simulink model "MdSWReqChk"  (R2024b)
settings: Solver=FixedStepDiscrete  StartTime=0.0  StopTime=10.0  FixedStep=0.01  RelTol=1e-3
undefined symbols (not defined in the file or in its folder): ChkBsyBitArray4s, ChkBsyBitArray6s7s, KeSMSAutoEZEFwdBkwdPosEna_Val, KeSMSuButtonLongPressedThrshldTm_Val, KeSMSuMdNum4s_Val, KeSMSuMdNum6s7s_Val, SetBsyBitArray4s, SetEnBitArray4s
libraries: simulink x16, RspLib x14
(part 2 of 3)

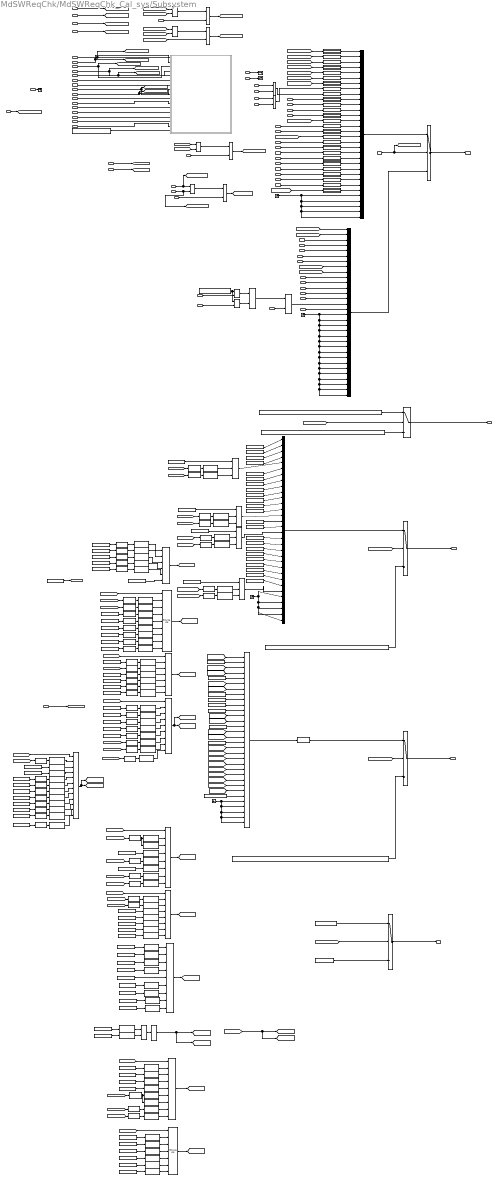
== system MdSWReqChk/MdSWReqChk_Cal_sys/Subsystem ==
  note: 0000 0010 1100 1101 1110 0000 0111 1000
  note: 2023.12.28 迎宾向后，条件改为或
  note: bug542961
  note: 符号方向反了，<= 改为>=
  note: 2023.8.1 CR401790 增加模式21-26的请求
  note: VIPR
  note: RcvyR
  note: VIPR
  note: LugL
  note: LugL
  note: LugR
  note: LugL
  note: LugL
  note: LugL
  note: LugR
  note: VIPR
  note: Md57
  note: Md57
  note: Md57
  note: LugR
  note: bedr
  acsEntyMdReq_Val_read : Inport
  acsExtMdReq_Val_read : Inport  Port=2
  AllLugMdReq_Val_read : Inport  Port=3
  AllVipMdReq_Val_read : Inport  Port=4
  EZE4sLtMdReq_Val_read : Inport  Port=5
  EZE4sRtMdReq_Val_read : Inport  Port=6
  EZQ4sLtMdReq_Val_read : Inport  Port=7
  EZQ4sRtMdReq_Val_read : Inport  Port=8
  IntimacyRtMdReq_Val_read : Inport  Port=9
  INTMMdReq_Val_read : Inport  Port=10
  LfFamlyReq_Val_read : Inport  Port=11
  LfLyMdReq_Val_read : Inport  Port=12
  LgrstCloseLtMdReq_Val_read : Inport  Port=13
  LgrstCloseRtMdReq_Val_read : Inport  Port=14
  LgrstOpenLtMdReq_Val_read : Inport  Port=15
  LgrstOpenRtMdReq_Val_read : Inport  Port=16
  LtLugMdReq_Val_read : Inport  Port=17
  LtRcvyMdReq_Val_read : Inport  Port=18
  LtVipMdReq_Val_read : Inport  Port=19
  LugMdLtAvl_Val_read : Inport  Port=20
  LugMdRtAvl_Val_read : Inport  Port=21
  MdSWIntSrc_R_Val_read : Inport  Port=22
  RtFamlyMdReq_Val_read : Inport  Port=23
  RtLugMdReq_Val_read : Inport  Port=24
  RtLyMdReq_Val_read : Inport  Port=25
  RtRcvyMdReq_Val_read : Inport  Port=26
  RtVipMdReq_Val_read : Inport  Port=27
  StNumFlg_Is4s_read : Inport  Port=28
  StNumFlg_Is6s_read : Inport  Port=29
  StNumFlg_Is6s7s_read : Inport  Port=30
  StNumFlg_Is7s_read : Inport  Port=31
  SwIntAcsEnty_Val_read : Inport  Port=32
  SwIntAcsExt_Val_read : Inport  Port=33
  SwIntAllLug_Val_read : Inport  Port=34
  SwIntLfRcvy_Val_read : Inport  Port=35
  SwIntLfVip_Val_read : Inport  Port=36
  SwIntRtRcvy_Val_read : Inport  Port=37
  SwIntRtVip_Val_read : Inport  Port=38
  VipMdLtAvl_Val_read : Inport  Port=39
  VipMdRtAvl_Val_read : Inport  Port=40
  WelcomeBkwdMdReq_Val_read : Inport  Port=41
  WelcomeFwdMdReq_Val_read : Inport  Port=42
  modestate32 : Inport  Port=43
  IfVeSMSuSecRwLtStFrwdBkwdPos_Val_read : Inport  Port=44
  IfVeSMSuSecRwRtStFrwdBkwdPos_Val_read : Inport  Port=45
  Md27Req_Val_read : Inport  Port=46
  Md28Req_Val_read : Inport  Port=47
  Md30Req_Val_read : Inport  Port=48
  Md31Req_Val_read : Inport  Port=49
  Md32Req_Val_read : Inport  Port=50
  Md53Req_Val_read : Inport  Port=51
  Md29Req_Val_read : Inport  Port=52
  VipExitMdLtAvl_Val_read : Inport  Port=53
  VipExitMdRtAvl_Val_read : Inport  Port=54
  Md56Req_Val_read : Inport  Port=55
  Md57Req_Val_read : Inport  Port=56
  Md58Req_Val_read : Inport  Port=57
  Md62Req_Val_read : Inport  Port=58
  Md61Req_Val_read : Inport  Port=59
  Md61MemReq_Val_read : Inport  Port=60
  Md62MemReq_Val_read : Inport  Port=61
  BigBedAllMdReq_Val_read : Inport  Port=62
  BigBedLMdAvl_Val_read : Inport  Port=63
  BigBedLtMdReq_Val_read : Inport  Port=64
  BigBedRMdAvl_Val_read : Inport  Port=65
  BigBedRtMdReq_Val_read : Inport  Port=66
  Bitwise Operator{,1,6,15} (4 alike) : simulink/Logic and Bit Operations/Bitwise Operator  logicop=OR  UseBitMask=off  NumInputPorts=3  BitMask=bin2dec('11011001')  BitMaskRealWorld=Stored Integer
  Bitwise Operator10 : simulink/Logic and Bit Operations/Bitwise Operator  logicop=OR  UseBitMask=off  NumInputPorts=7  BitMask=bin2dec('11011001')  BitMaskRealWorld=Stored Integer
  Bitwise Operator{2,8..9,11} (4 alike) : simulink/Logic and Bit Operations/Bitwise Operator  logicop=OR  UseBitMask=off  NumInputPorts=9  BitMask=bin2dec('11011001')  BitMaskRealWorld=Stored Integer
  Bitwise Operator12 : simulink/Logic and Bit Operations/Bitwise Operator  logicop=OR  UseBitMask=off  NumInputPorts=7  BitMask=bin2dec('11011001')  BitMaskRealWorld=Stored Integer
  Bitwise Operator13 : simulink/Logic and Bit Operations/Bitwise Operator  logicop=OR  UseBitMask=off  NumInputPorts=2  BitMask=bin2dec('11011001')  BitMaskRealWorld=Stored Integer
  Bitwise Operator14 : simulink/Logic and Bit Operations/Bitwise Operator  logicop=NOT  UseBitMask=off  BitMask=bin2dec('11011001')  BitMaskRealWorld=Stored Integer
  Bitwise Operator3 : simulink/Logic and Bit Operations/Bitwise Operator  logicop=OR  UseBitMask=off  NumInputPorts=12  BitMask=bin2dec('11011001')  BitMaskRealWorld=Stored Integer
  Bitwise Operator4 : simulink/Logic and Bit Operations/Bitwise Operator  logicop=OR  UseBitMask=off  NumInputPorts=8  BitMask=bin2dec('11011001')  BitMaskRealWorld=Stored Integer
  Bitwise Operator5 : simulink/Logic and Bit Operations/Bitwise Operator  logicop=OR  UseBitMask=off  NumInputPorts=8  BitMask=bin2dec('11011001')  BitMaskRealWorld=Stored Integer
  Bitwise Operator7 : simulink/Logic and Bit Operations/Bitwise Operator  logicop=OR  UseBitMask=off  NumInputPorts=6  BitMask=bin2dec('11011001')  BitMaskRealWorld=Stored Integer
  Constant : Constant  Value=ChkBsyBitArray6s7s  OutDataTypeStr=uint32
  Constant1 : Constant  Value=ChkBsyBitArray4s  OutDataTypeStr=uint32
  Constant10 : Constant  Value=268435456  OutDataTypeStr=uint32
  Constant101 : Constant  Value=0xffffffff  OutDataTypeStr=uint32
  Constant{19..20,24..25,39..44,47,50..55,57..60,62..66,68..92,94,102} (53 alike) : Constant  OutDataTypeStr=uint32
  Constant{11..18} (8 alike) : Constant  Value=4294967295  OutDataTypeStr=uint32
  Constant2 : Constant  Value=SetEnBitArray4s  OutDataTypeStr=uint32
  Constant21 : Constant  Value=1048576  OutDataTypeStr=uint32
  Constant22 : Constant  Value=2097152  OutDataTypeStr=uint32
  Constant{23,45..46,48..49,61,67,93} (8 alike) : Constant  Value=0  OutDataTypeStr=uint32
  Constant26 : Constant  Value=8  OutDataTypeStr=uint32
  Constant27 : Constant  Value=512  OutDataTypeStr=uint32
  Constant28 : Constant  Value=2048  OutDataTypeStr=uint32
  Constant29 : Constant  Value=2  OutDataTypeStr=uint32
  Constant3 : Constant  Value=67108864  OutDataTypeStr=uint32
  Constant30 : Constant  Value=1024  OutDataTypeStr=uint32
  Constant31 : Constant  Value=4096  OutDataTypeStr=uint32
  Constant32 : Constant  Value=64  OutDataTypeStr=uint32
  Constant33 : Constant  Value=32  OutDataTypeStr=uint32
  Constant34 : Constant  Value=16  OutDataTypeStr=uint32
  Constant35 : Constant  Value=524288  OutDataTypeStr=uint32
  Constant36 : Constant  Value=128  OutDataTypeStr=uint32
  Constant37 : Constant  Value=256  OutDataTypeStr=uint32
  Constant38 : Constant  Value=4  OutDataTypeStr=uint32
  Constant4 : Constant  Value=134217728  OutDataTypeStr=uint32
  Constant5 : Constant  Value=536870912  OutDataTypeStr=uint32
  Constant56 : Constant  Value=16777216  OutDataTypeStr=uint32
  Constant6 : Constant  Value=1073741824  OutDataTypeStr=uint32
  Constant7 : Constant  Value=SetBsyBitArray4s  OutDataTypeStr=uint32
  Constant8 : Constant  Value=2147483648  OutDataTypeStr=uint32
  Constant9 : Constant  Value=131072  OutDataTypeStr=uint32
  Constant95 : Constant  Value=8192  OutDataTypeStr=uint32
  Constant96 : Constant  Value=16384  OutDataTypeStr=uint32
  Constant98 : Constant  Value=32768  OutDataTypeStr=uint32
  Data Type Conversion{,1..10,12..51,53..54} (53 alike) : DataTypeConversion  OutDataTypeStr=uint32  SaturateOnIntegerOverflow=off  RndMeth=Floor
  Data Type Conversion11 : DataTypeConversion  SaturateOnIntegerOverflow=off  RndMeth=Floor
  Ground{,1..3} (4 alike) : Ground
  Logical Operator{,2,4,6,8..10} (7 alike) : Logic  Operator=OR  AllPortsSameDT=off  OutDataTypeStr=boolean
  Logical Operator{1,3,5,7,11} (5 alike) : Logic  AllPortsSameDT=off  OutDataTypeStr=boolean
  Mux{,1..3} (4 alike) : Mux  Inputs=32
  NotUsedMode : Constant  Value=47046776  OutDataTypeStr=uint32
  PA_KeSMSAutoEZEFwdBkwdPosEna_Val : Constant  Value=KeSMSAutoEZEFwdBkwdPosEna_Val
  PA_KeSMSuButtonLongPressedThrshldTm_Val : Constant  Value=KeSMSuButtonLongPressedThrshldTm_Val
  PA_KeSMSuMdNum4s_Val : Constant  Value=KeSMSuMdNum4s_Val
  PA_KeSMSuMdNum6s7s_Val : Constant  Value=KeSMSuMdNum6s7s_Val
  Relational Operator : RelationalOperator  OutDataTypeStr=boolean  RndMeth=Simplest  InputSameDT=off
  Relational Operator1 : RelationalOperator  OutDataTypeStr=boolean  RndMeth=Simplest  InputSameDT=off
  ReqTrig : Subsystem
  ReqTrig1 : Subsystem
  ReqTrig10 : Subsystem
  ReqTrig11 : Subsystem
  ReqTrig12 : Subsystem
  ReqTrig13 : Subsystem
  ReqTrig14 : Subsystem
  ReqTrig15 : Subsystem
  ReqTrig16 : Subsystem
  ReqTrig17 : Subsystem
  ReqTrig18 : Subsystem
  ReqTrig19 : Subsystem
  ReqTrig2 : Subsystem
  ReqTrig20 : Subsystem
  ReqTrig21 : Subsystem
  ReqTrig22 : Subsystem
  ReqTrig23 : Subsystem
  ReqTrig24 : Subsystem
  ReqTrig25 : Subsystem
  ReqTrig26 : Subsystem
  ReqTrig3 : Subsystem
  ReqTrig4 : Subsystem
  ReqTrig5 : Subsystem
  ReqTrig6 : Subsystem
  ReqTrig7 : Subsystem
  ReqTrig8 : Subsystem
  ReqTrig9 : Subsystem
  Shift Arithmetic{,27,44,52} (4 alike) : ArithShift  BitShiftNumber=9  BitShiftDirection=Left
  Shift Arithmetic{1,8..9,20,45,55,58} (7 alike) : ArithShift  BitShiftNumber=11  BitShiftDirection=Left
  Shift Arithmetic10 : ArithShift  BitShiftNumber=26  BitShiftDirection=Left
  Shift Arithmetic{11,26,36,39} (4 alike) : ArithShift  BitShiftNumber=27  BitShiftDirection=Left
  Shift Arithmetic12 : ArithShift  BitShiftNumber=29  BitShiftDirection=Left
  Shift Arithmetic13 : ArithShift  BitShiftNumber=30  BitShiftDirection=Left
  Shift Arithmetic{14,28,33,50} (4 alike) : ArithShift  BitShiftNumber=31  BitShiftDirection=Left
  Shift Arithmetic{3,15,23..24,47,57} (6 alike) : ArithShift  BitShiftNumber=8  BitShiftDirection=Left
  Shift Arithmetic16 : ArithShift  BitShiftDirection=Left
  Shift Arithmetic17 : ArithShift  BitShiftNumber=1  BitShiftDirection=Left
  Shift Arithmetic18 : ArithShift  BitShiftNumber=2  BitShiftDirection=Left
  Shift Arithmetic19 : ArithShift  BitShiftNumber=24  BitShiftDirection=Left
  Shift Arithmetic{2,5,22,25,31,46,51} (7 alike) : ArithShift  BitShiftNumber=7  BitShiftDirection=Left
  Shift Arithmetic{21,35,38,40,56} (5 alike) : ArithShift  BitShiftNumber=17  BitShiftDirection=Left
  Shift Arithmetic29 : ArithShift  BitShiftNumber=26  BitShiftDirection=Left
  Shift Arithmetic30 : ArithShift  BitShiftNumber=28  BitShiftDirection=Left
  Shift Arithmetic32 : ArithShift  BitShiftNumber=10  BitShiftDirection=Left
  Shift Arithmetic34 : ArithShift  BitShiftNumber=26  BitShiftDirection=Left
  Shift Arithmetic37 : ArithShift  BitShiftNumber=13  BitShiftDirection=Left
  Shift Arithmetic{4,6..7,42,54,59} (6 alike) : ArithShift  BitShiftNumber=12  BitShiftDirection=Left
  Shift Arithmetic41 : ArithShift  BitShiftNumber=1  BitShiftDirection=Left
  Shift Arithmetic43 : ArithShift  BitShiftNumber=10  BitShiftDirection=Left
  Shift Arithmetic48 : ArithShift  BitShiftNumber=29  BitShiftDirection=Left
  Shift Arithmetic49 : ArithShift  BitShiftNumber=30  BitShiftDirection=Left
  Shift Arithmetic53 : ArithShift  BitShiftNumber=10  BitShiftDirection=Left
  Shift Arithmetic{60,62,64,66,68,70,72,74} (8 alike) : ArithShift  BitShiftNumber=20  BitShiftDirection=Left
  Shift Arithmetic{61,63,65,67,69,71,73,75} (8 alike) : ArithShift  BitShiftNumber=21  BitShiftDirection=Left
  Shift Arithmetic76 : ArithShift  BitShiftNumber=29  BitShiftDirection=Left
  Shift Arithmetic77 : ArithShift  BitShiftNumber=30  BitShiftDirection=Left
  Shift Arithmetic78 : ArithShift  BitShiftNumber=14  BitShiftDirection=Left
  Shift Arithmetic80 : ArithShift  BitShiftNumber=14  BitShiftDirection=Left
  Shift Arithmetic81 : ArithShift  BitShiftNumber=13  BitShiftDirection=Left
  Subsystem : Subsystem  Commented=on
  Switch{,1..4} (5 alike) : Switch  Criteria=u2 > Threshold  SaturateOnIntegerOverflow=off  InputSameDT=off
  Terminator : Terminator
  Terminator1 : Terminator
  Terminator_28 : Terminator
  VIPR : ArithShift  BitShiftNumber=11  BitShiftDirection=Left
  VIPR1 : ArithShift  BitShiftNumber=27  BitShiftDirection=Left
  VIPR2 : ArithShift  BitShiftNumber=28  BitShiftDirection=Left
  ChkBsyBitArray_Val_write : Outport  VectorParamsAs1DForOutWhenUnconnected=off
      settings: EnsureOutportIsVirtual=on
  MdReqArray_Val_write : Outport  Port=2  VectorParamsAs1DForOutWhenUnconnected=off
      settings: EnsureOutportIsVirtual=on
  SetBsyBitArray_Val_write : Outport  Port=3  VectorParamsAs1DForOutWhenUnconnected=off
      settings: EnsureOutportIsVirtual=on
  SetEnBitArray_Val_write : Outport  Port=4  VectorParamsAs1DForOutWhenUnconnected=off
      settings: EnsureOutportIsVirtual=on
  VeSMSuMdNum_Val_write : Outport  Port=5  VectorParamsAs1DForOutWhenUnconnected=off
      settings: EnsureOutportIsVirtual=on
  wires:
  StNumFlg_Is4s_read/1 -> Terminator_28/1
  StNumFlg_Is7s_read/1 -> [is7s]
  PA_KeSMSuButtonLongPressedThrshldTm_Val/1 -> Subsystem/17(KeSMSuButtonLongPressedThrshldTm_Val)
  StNumFlg_Is6s_read/1 -> [Is6s]
  modestate32/1 -> Subsystem/7(modestate32_Val_read)
  acsEntyMdReq_Val_read/1 -> [EZEReq], Subsystem/1(acsEntyMdReq_Val_read)
  AllLugMdReq_Val_read/1 -> [AllLugReq], Subsystem/3(AllLugMdReq_Val_read)
  acsExtMdReq_Val_read/1 -> [EZQReq], Subsystem/2(acsExtMdReq_Val_read)
  MdSWIntSrc_R_Val_read/1 -> Subsystem/6(MdSWIntSrc_R_Val_read)
  LtVipMdReq_Val_read/1 -> [LtVIPReq], Subsystem/5(LtVipMdReq_Val_read)
  LtRcvyMdReq_Val_read/1 -> [LtRcvyReq], Subsystem/4(LtRcvyMdReq_Val_read)
  RtRcvyMdReq_Val_read/1 -> [RtRcvyReq], Subsystem/8(RtRcvyMdReq_Val_read)
  RtVipMdReq_Val_read/1 -> [RtVIPReq], Subsystem/9(RtVipMdReq_Val_read)
  SwIntAcsEnty_Val_read/1 -> Subsystem/10(SwIntAcsEnty_Val_read)
  SwIntAcsExt_Val_read/1 -> Subsystem/11(SwIntAcsExt_Val_read)
  SwIntLfRcvy_Val_read/1 -> Subsystem/12(SwIntLfRcvy_Val_read)
  SwIntLfVip_Val_read/1 -> Subsystem/13(SwIntLfVip_Val_read)
  SwIntRtVip_Val_read/1 -> Subsystem/15(SwIntRtVip_Val_read)
  SwIntAllLug_Val_read/1 -> Subsystem/16(SwIntAllLug_Val_read)
  SwIntRtRcvy_Val_read/1 -> Subsystem/14(SwIntRtRcvy_Val_read)
  [EZEReq] -> ReqTrig/1(Req)
  [EZQReq] -> ReqTrig1/1(Req)
  [LtVIPReq] -> ReqTrig2/1(Req)
  [RtVIPReq] -> ReqTrig3/1(Req)
  VipMdLtAvl_Val_read/1 -> [VipLtAvl]
  VipMdRtAvl_Val_read/1 -> [VipRtAvl]
  [VipLtAvl] -> Logical Operator/1
  [VipRtAvl] -> Logical Operator/2
  Logical Operator/1 -> Logical Operator1/1
  AllVipMdReq_Val_read/1 -> Logical Operator1/2
  Logical Operator1/1 -> [AllVipReq]
  [AllVipReq] -> ReqTrig4/1(Req)
  [LtRcvyReq] -> ReqTrig5/1(Req)
  [RtRcvyReq] -> ReqTrig6/1(Req)
  INTMMdReq_Val_read/1 -> ReqTrig9/1(Req)
  IntimacyRtMdReq_Val_read/1 -> ReqTrig10/1(Req)
  LtLugMdReq_Val_read/1 -> ReqTrig11/1(Req)
  RtLugMdReq_Val_read/1 -> ReqTrig12/1(Req)
  Logical Operator3/1 -> [AllLugReqComfirm]
  [AllLugReq] -> Logical Operator3/2
  Logical Operator2/1 -> Logical Operator3/1
  LugMdLtAvl_Val_read/1 -> [LugLtAvl]
  LugMdRtAvl_Val_read/1 -> [LugRtAvl]
  [LugLtAvl] -> Logical Operator2/1
  [LugRtAvl] -> Logical Operator2/2
  [AllLugReqComfirm] -> ReqTrig13/1(Req)
  Switch/1 -> MdReqArray_Val_write/1
  StNumFlg_Is6s7s_read/1 -> [Is6s7s], Switch/2
  Mux/1 -> Switch/1
  [LtVIPReq] -> Mux1/1
  [LtRcvyReq] -> Mux1/2
  LfLyMdReq_Val_read/1 -> Mux1/3
  LgrstOpenLtMdReq_Val_read/1 -> Mux1/4
  LgrstCloseLtMdReq_Val_read/1 -> Mux1/5
  [RtVIPReq] -> Mux1/8
  [RtRcvyReq] -> Mux1/9
  RtLyMdReq_Val_read/1 -> Mux1/10
  LgrstOpenRtMdReq_Val_read/1 -> Mux1/11
  LgrstCloseRtMdReq_Val_read/1 -> Mux1/12
  EZE4sRtMdReq_Val_read/1 -> Mux1/13
  EZQ4sRtMdReq_Val_read/1 -> Mux1/14
  WelcomeFwdMdReq_Val_read/1 -> Mux1/16
  Ground1/1 -> Mux1/27, Mux1/28, Mux1/32, Mux1/31, Mux1/30, Mux1/29, Mux1/26, Mux1/25, Mux1/24, Mux1/23, Mux1/22, Mux1/21, Mux1/20, Mux1/19, Mux1/18, Mux1/17
  Mux1/1 -> Switch/3
  [Is6s7s] -> Switch1/2
  Switch1/1 -> ChkBsyBitArray_Val_write/1
  Constant/1 -> Switch1/1
  Constant1/1 -> Switch1/3
  Constant2/1 -> Switch2/3
  [Is6s7s] -> Switch2/2
  Constant33/1 -> Mux2/9
  Mux2/1 -> Switch2/1  "SetEnBitArray"
  Data Type Conversion/1 -> Shift Arithmetic/1
  Constant37/1 -> Mux2/13
  Constant39/1 -> Mux2/1
  [VipRtAvl] -> Data Type Conversion1/1
  Constant28/1 -> Mux2/4
  Constant26/1 -> Mux2/2
  Bitwise Operator/1 -> Mux2/5
  Constant32/1 -> Mux2/8
  Constant30/1 -> Mux2/6
  Bitwise Operator1/1 -> Mux2/14
  Constant35/1 -> Mux2/11
  [VipLtAvl] -> Data Type Conversion/1
  Constant31/1 -> Mux2/7
  Constant34/1 -> Mux2/10
  Constant36/1 -> Mux2/12
  Constant29/1 -> Bitwise Operator/1
  [LugLtAvl] -> Data Type Conversion2/1
  Shift Arithmetic/1 -> Bitwise Operator/2
  Constant27/1 -> Mux2/3
  Data Type Conversion1/1 -> Shift Arithmetic1/1
  Constant38/1 -> Bitwise Operator1/1
  Shift Arithmetic1/1 -> Bitwise Operator/3
  Data Type Conversion2/1 -> Shift Arithmetic2/1
  Shift Arithmetic2/1 -> Bitwise Operator1/2
  [LugRtAvl] -> Data Type Conversion3/1
  Data Type Conversion3/1 -> Shift Arithmetic3/1
  Shift Arithmetic3/1 -> Bitwise Operator1/3
  Switch2/1 -> SetEnBitArray_Val_write/1
  Switch3/1 -> SetBsyBitArray_Val_write/1
  [Is6s7s] -> Switch3/2
  Constant7/1 -> Switch3/3
  Constant12/1 -> Mux3/5
  Constant16/1 -> Mux3/10
  Data Type Conversion11/1 -> Switch3/1  "SetBsyBitArray"
  Constant15/1 -> Mux3/9
  Constant14/1 -> Mux3/8
  [BsyBitEZE] -> Mux3/1
  [RghtBsyBitLug] -> Mux3/13
  Constant17/1 -> Mux3/11
  [RghtBsyBitRcvy] -> Mux3/7
  Constant11/1 -> Mux3/2
  [LftBsyBitVIP] -> Mux3/3
  [LftBsyBitLug] -> Mux3/12
  Mux3/1 -> Data Type Conversion11/1
  [RghtBsyBitVIP] -> Mux3/4
  [LftBsyBitRcvy] -> Mux3/6
  [is7s] -> Data Type Conversion5/1
  Shift Arithmetic8/1 -> Bitwise Operator4/3
  [BsyAll] -> Bitwise Operator4/1
  [is7s] -> Data Type Conversion7/1
  [is7s] -> Data Type Conversion6/1
  Shift Arithmetic9/1 -> Bitwise Operator5/2
  [BsyAll] -> Bitwise Operator5/1
  Bitwise Operator3/1 -> [RghtBsyBitVIP], [VIPRExitBsyBit]
  Data Type Conversion7/1 -> Shift Arithmetic9/1
  Bitwise Operator4/1 -> [LftBsyBitLug]
  Shift Arithmetic6/1 -> Bitwise Operator4/2
  Data Type Conversion5/1 -> Shift Arithmetic5/1
  [BsyAll] -> Bitwise Operator2/1
  Data Type Conversion6/1 -> Shift Arithmetic8/1, Shift Arithmetic6/1
  Bitwise Operator5/1 -> [RghtBsyBitLug]
  Shift Arithmetic5/1 -> Bitwise Operator3/2
  Bitwise Operator2/1 -> [LftBsyBitVIP], [VIPLExitBsyBit]
  [BsyAll] -> Bitwise Operator3/1
  [Is6s7s] -> Switch4/2
  PA_KeSMSuMdNum4s_Val/1 -> Switch4/3
  PA_KeSMSuMdNum6s7s_Val/1 -> Switch4/1  "SetBsyBitArray"
  Switch4/1 -> VeSMSuMdNum_Val_write/1
  PA_KeSMSAutoEZEFwdBkwdPosEna_Val/1 -> Relational Operator1/1, Relational Operator/1
  IfVeSMSuSecRwLtStFrwdBkwdPos_Val_read/1 -> Relational Operator/2
  IfVeSMSuSecRwRtStFrwdBkwdPos_Val_read/1 -> Relational Operator1/2
  Relational Operator/1 -> Logical Operator4/1
  Relational Operator1/1 -> Logical Operator4/2
  Logical Operator5/1 -> Mux1/15
  WelcomeBkwdMdReq_Val_read/1 -> Logical Operator5/2
  Logical Operator4/1 -> Logical Operator5/1
  Md27Req_Val_read/1 -> ReqTrig14/1(Req)
  Md28Req_Val_read/1 -> ReqTrig15/1(Req)
  Constant3/1 -> Mux2/15
  Constant4/1 -> Mux2/16
  [Md29Req] -> ReqTrig16/1(Req)
  Md32Req_Val_read/1 -> ReqTrig19/1(Req)
  Md53Req_Val_read/1 -> ReqTrig20/1(Req)
  Constant5/1 -> Mux2/18
  Constant6/1 -> Mux2/19
  Constant8/1 -> Mux2/20
  Bitwise Operator6/1 -> Mux2/17
  Constant10/1 -> Bitwise Operator6/1
  Shift Arithmetic10/1 -> Bitwise Operator6/2
  Data Type Conversion8/1 -> Shift Arithmetic10/1
  [VIPLExittAvl] -> Data Type Conversion8/1
  [VIPRExittAvl] -> Data Type Conversion9/1
  Data Type Conversion9/1 -> Shift Arithmetic11/1
  Shift Arithmetic11/1 -> Bitwise Operator6/3
  Constant13/1 -> Mux3/14
  [VIPLExitBsyBit] -> Mux3/15
  [VIPRExitBsyBit] -> Mux3/16
  Constant18/1 -> Mux3/17
  [BsyBitThdExpandL] -> Mux3/20
  [BsyBitThdExpandR] -> Mux3/21
  Constant41/1 -> Shift Arithmetic12/1
  Constant43/1 -> Shift Arithmetic13/1
  Shift Arithmetic12/1 -> Bitwise Operator3/3
  Shift Arithmetic13/1 -> Bitwise Operator3/4
  Shift Arithmetic14/1 -> Bitwise Operator4/4
  Constant44/1 -> Shift Arithmetic14/1
  [BsyBitPass] -> Mux3/18
  [BsyBitPass] -> Mux3/19
  [BsyAll] -> Bitwise Operator9/1
  Shift Arithmetic22/1 -> Bitwise Operator9/2
  Data Type Conversion12/1 -> Shift Arithmetic22/1
  Bitwise Operator9/1 -> [RghtBsyBitRcvy]
  VipExitMdLtAvl_Val_read/1 -> [VIPLExittAvl]
  VipExitMdRtAvl_Val_read/1 -> [VIPRExittAvl]
  [VIPRExittAvl] -> Logical Operator6/2
  [VIPLExittAvl] -> Logical Operator6/1
  Logical Operator6/1 -> Logical Operator7/1
  Md29Req_Val_read/1 -> Logical Operator7/2
  Logical Operator7/1 -> [Md29Req]
  [is7s] -> Data Type Conversion12/1
  Bitwise Operator10/1 -> [LftBsyBitRcvy]
  [BsyAll] -> Bitwise Operator10/1
  Constant23/1 -> Data Type Conversion13/1
  Data Type Conversion13/1 -> Shift Arithmetic23/1
  Shift Arithmetic23/1 -> Bitwise Operator10/2
  Shift Arithmetic24/1 -> Bitwise Operator9/3  "LugR"
  Data Type Conversion14/1 -> Shift Arithmetic24/1
  [is7s] -> Data Type Conversion14/1
  Shift Arithmetic25/1 -> Bitwise Operator10/3
  Data Type Conversion15/1 -> Shift Arithmetic25/1
  [is7s] -> Data Type Conversion15/1
  Md56Req_Val_read/1 -> ReqTrig21/1(Req)
  [BsyBitBigFourSt] -> Mux3/22
  Md30Req_Val_read/1 -> ReqTrig17/1(Req)
  Md31Req_Val_read/1 -> ReqTrig18/1(Req)
  Constant51/1 -> VIPR/1
  Constant47/1 -> Data Type Conversion16/1
  Data Type Conversion16/1 -> Shift Arithmetic16/1
  Constant48/1 -> Data Type Conversion17/1
  Data Type Conversion17/1 -> Shift Arithmetic17/1
  Data Type Conversion18/1 -> Shift Arithmetic18/1
  Constant49/1 -> Data Type Conversion18/1
  Bitwise Operator7/1 -> [BsyAll]
  Constant50/1 -> Data Type Conversion19/1
  Data Type Conversion19/1 -> Shift Arithmetic19/1
  Constant52/1 -> Data Type Conversion20/1
  Data Type Conversion20/1 -> Shift Arithmetic20/1
  Data Type Conversion21/1 -> Shift Arithmetic21/1
  Constant53/1 -> Data Type Conversion21/1
  Constant54/1 -> Data Type Conversion22/1
  Data Type Conversion22/1 -> Shift Arithmetic26/1
  Shift Arithmetic20/1 -> Bitwise Operator9/4  "VIPR"
  Shift Arithmetic21/1 -> Bitwise Operator9/5  "Md53"
  Shift Arithmetic26/1 -> Bitwise Operator9/6  "Md28"
  Data Type Conversion24/1 -> Shift Arithmetic28/1
  Constant58/1 -> Data Type Conversion23/1
  Constant59/1 -> Data Type Conversion24/1
  Shift Arithmetic28/1 -> Bitwise Operator10/5  "ExpandL"
  Shift Arithmetic27/1 -> Bitwise Operator10/4  "VIPL"
  Data Type Conversion25/1 -> Shift Arithmetic29/1
  Constant60/1 -> Data Type Conversion25/1
  Shift Arithmetic29/1 -> Bitwise Operator10/6  "VIPLExit"
  Data Type Conversion23/1 -> Shift Arithmetic27/1
  Data Type Conversion26/1 -> Shift Arithmetic30/1
  Constant61/1 -> Data Type Conversion26/1
  Constant82/1 -> Data Type Conversion27/1
  Shift Arithmetic31/1 -> Bitwise Operator2/2
  Data Type Conversion27/1 -> Shift Arithmetic31/1
  Shift Arithmetic32/1 -> Bitwise Operator2/3  "RcvyL"
  Shift Arithmetic33/1 -> Bitwise Operator2/4  "ExpandL"
  Data Type Conversion28/1 -> Shift Arithmetic32/1
  Data Type Conversion29/1 -> Shift Arithmetic33/1
  Shift Arithmetic34/1 -> Bitwise Operator2/5  "VIPLExit"
  Constant62/1 -> Data Type Conversion30/1
  Data Type Conversion30/1 -> Shift Arithmetic34/1
  Constant55/1 -> Data Type Conversion29/1
  Constant42/1 -> Data Type Conversion28/1
  Data Type Conversion31/1 -> Shift Arithmetic35/1
  Data Type Conversion4/1 -> Shift Arithmetic4/1
  Shift Arithmetic35/1 -> Bitwise Operator3/6  "ExpandR"
  Data Type Conversion32/1 -> Shift Arithmetic36/1
  Constant64/1 -> Data Type Conversion31/1
  Shift Arithmetic4/1 -> Bitwise Operator3/5  "RcvyR"
  Constant63/1 -> Data Type Conversion4/1
  Constant65/1 -> Data Type Conversion32/1
  Shift Arithmetic36/1 -> Bitwise Operator3/7  "VIPRExit"
  Shift Arithmetic7/1 -> Bitwise Operator5/3  "RcvyR"
  Shift Arithmetic16/1 -> Bitwise Operator7/1
  Shift Arithmetic17/1 -> Bitwise Operator7/2
  Shift Arithmetic18/1 -> Bitwise Operator7/3
  Shift Arithmetic19/1 -> Bitwise Operator7/4
  Shift Arithmetic30/1 -> Bitwise Operator7/5
  Shift Arithmetic38/1 -> Bitwise Operator4/5
  [is7s] -> Data Type Conversion33/1
  Data Type Conversion10/1 -> Shift Arithmetic7/1
  [is7s] -> Data Type Conversion10/1
  Shift Arithmetic39/1 -> Bitwise Operator5/4
  Constant24/1 -> Shift Arithmetic39/1
  Constant25/1 -> Shift Arithmetic40/1
  Shift Arithmetic40/1 -> Bitwise Operator5/5
  Bitwise Operator8/1 -> [BsyBitPass]
  VIPR/1 -> Bitwise Operator8/2
  Shift Arithmetic41/1 -> Bitwise Operator8/1
  Constant46/1 -> Shift Arithmetic41/1
  Constant66/1 -> VIPR1/1
  VIPR1/1 -> Bitwise Operator8/3
  VIPR2/1 -> Bitwise Operator8/4
  Constant67/1 -> VIPR2/1
  NotUsedMode/1 -> [NotUsedMode]
  Constant93/1 -> Bitwise Operator8/5
  Data Type Conversion33/1 -> Shift Arithmetic38/1
  Shift Arithmetic42/1 -> Bitwise Operator9/7  "RcvyR"
  Data Type Conversion34/1 -> Shift Arithmetic42/1
  Constant19/1 -> Data Type Conversion34/1
  Data Type Conversion35/1 -> Shift Arithmetic43/1
  Shift Arithmetic43/1 -> Bitwise Operator10/7  "RcvyL"
  Constant20/1 -> Data Type Conversion35/1
  Data Type Conversion36/1 -> Shift Arithmetic44/1
  Shift Arithmetic44/1 -> Bitwise Operator2/6  "VIPL"
  Constant68/1 -> Data Type Conversion36/1
  Shift Arithmetic45/1 -> Bitwise Operator3/8  "VIPR"
  Data Type Conversion37/1 -> Shift Arithmetic45/1
  Constant69/1 -> Data Type Conversion37/1
  Constant70/1 -> Shift Arithmetic46/1
  Shift Arithmetic46/1 -> Bitwise Operator4/6
  Shift Arithmetic47/1 -> Bitwise Operator5/6
  Constant71/1 -> Shift Arithmetic47/1
  Shift Arithmetic48/1 -> Bitwise Operator8/6
  Constant72/1 -> Shift Arithmetic48/1
  Constant73/1 -> Shift Arithmetic49/1
  Shift Arithmetic49/1 -> Bitwise Operator8/7
  Bitwise Operator14/1 -> [BsyBitBigFourSt], [BsyBitEZE]
  [BsyAll] -> Bitwise Operator11/1
  Bitwise Operator11/1 -> [BsyBitThdExpandL]
  Constant40/1 -> Shift Arithmetic50/1
  Shift Arithmetic50/1 -> Bitwise Operator11/2
  Constant57/1 -> Shift Arithmetic51/1
  Shift Arithmetic51/1 -> Bitwise Operator11/3
  Shift Arithmetic52/1 -> Bitwise Operator11/4
  Constant74/1 -> Shift Arithmetic52/1
  Shift Arithmetic53/1 -> Bitwise Operator11/5
  Constant75/1 -> Shift Arithmetic53/1
  Data Type Conversion38/1 -> Shift Arithmetic54/1, Shift Arithmetic55/1
  Shift Arithmetic54/1 -> Bitwise Operator11/6
  [is7s] -> Data Type Conversion38/1
  Shift Arithmetic55/1 -> Bitwise Operator11/7
  Bitwise Operator12/1 -> [BsyBitThdExpandR]
  Constant79/1 -> Shift Arithmetic59/1
  Shift Arithmetic59/1 -> Bitwise Operator12/5
  Constant78/1 -> Shift Arithmetic58/1
  Shift Arithmetic58/1 -> Bitwise Operator12/4
  Shift Arithmetic57/1 -> Bitwise Operator12/3
  Constant77/1 -> Shift Arithmetic57/1
  Shift Arithmetic56/1 -> Bitwise Operator12/2
  Constant76/1 -> Shift Arithmetic56/1
  [BsyAll] -> Bitwise Operator12/1
  EZE4sLtMdReq_Val_read/1 -> Mux1/6
  EZQ4sLtMdReq_Val_read/1 -> Mux1/7
  Md57Req_Val_read/1 -> ReqTrig22/1(Req)
  Md58Req_Val_read/1 -> ReqTrig23/1(Req)
  Constant9/1 -> Mux2/21
  Constant56/1 -> Mux2/22
  Constant22/1 -> Mux2/24
  Constant21/1 -> Mux2/23
  [BsyBitMd58] -> Mux3/24
  [BsyBitMd57] -> Mux3/23
  Constant80/1 -> Data Type Conversion39/1
  Data Type Conversion39/1 -> Shift Arithmetic60/1
  Shift Arithmetic60/1 -> Bitwise Operator9/8  "Md57"
  Shift Arithmetic61/1 -> Bitwise Operator9/9  "Md58"
  Data Type Conversion40/1 -> Shift Arithmetic61/1
  Constant81/1 -> Data Type Conversion40/1
  Shift Arithmetic62/1 -> Bitwise Operator2/7  "Md57"
  Data Type Conversion41/1 -> Shift Arithmetic62/1
  [is7s] -> Data Type Conversion41/1
  [is7s] -> Data Type Conversion42/1
  Data Type Conversion42/1 -> Shift Arithmetic63/1
  Shift Arithmetic63/1 -> Bitwise Operator2/8  "Md58"
  Constant83/1 -> Data Type Conversion43/1
  Data Type Conversion43/1 -> Shift Arithmetic64/1
  Shift Arithmetic64/1 -> Bitwise Operator3/9  "Md57"
  Shift Arithmetic65/1 -> Bitwise Operator3/10  "Md58"
  Data Type Conversion44/1 -> Shift Arithmetic65/1
  Constant84/1 -> Data Type Conversion44/1
  Shift Arithmetic66/1 -> Bitwise Operator4/7
  [is7s] -> Data Type Conversion45/1
  Data Type Conversion46/1 -> Shift Arithmetic67/1
  Shift Arithmetic67/1 -> Bitwise Operator4/8  "Md58"
  Data Type Conversion45/1 -> Shift Arithmetic66/1
  [is7s] -> Data Type Conversion46/1
  Shift Arithmetic69/1 -> Bitwise Operator5/8  "Md58"
  Shift Arithmetic68/1 -> Bitwise Operator5/7
  Constant85/1 -> Shift Arithmetic68/1
  Constant86/1 -> Shift Arithmetic69/1
  Constant88/1 -> Shift Arithmetic71/1
  Constant87/1 -> Shift Arithmetic70/1
  Shift Arithmetic70/1 -> Bitwise Operator8/8
  Shift Arithmetic71/1 -> Bitwise Operator8/9  "Md58"
  Shift Arithmetic72/1 -> Bitwise Operator11/8  "Md57"
  [is7s] -> Data Type Conversion47/1
  Data Type Conversion47/1 -> Shift Arithmetic72/1
  Data Type Conversion48/1 -> Shift Arithmetic73/1
  [is7s] -> Data Type Conversion48/1
  Shift Arithmetic73/1 -> Bitwise Operator11/9  "Md58"
  Constant89/1 -> Shift Arithmetic74/1
  Shift Arithmetic74/1 -> Bitwise Operator12/6
  Shift Arithmetic75/1 -> Bitwise Operator12/7
  Constant90/1 -> Shift Arithmetic75/1
  Shift Arithmetic77/1 -> Bitwise Operator13/2
  Constant92/1 -> Shift Arithmetic77/1
  Constant91/1 -> Shift Arithmetic76/1
  Shift Arithmetic76/1 -> Bitwise Operator13/1
  Bitwise Operator13/1 -> Bitwise Operator14/1
  [RghtBsyBitVIP] -> [BsyBitMd57], [BsyBitMd58]
  ReqTrig/1(ReqOut) -> Mux/1
  ReqTrig1/1(ReqOut) -> Mux/2
  ReqTrig2/1(ReqOut) -> Mux/3
  ReqTrig3/1(ReqOut) -> Mux/4
  ReqTrig4/1(ReqOut) -> Mux/5
  ReqTrig5/1(ReqOut) -> Mux/6
  ReqTrig6/1(ReqOut) -> Mux/7
  ReqTrig7/1(ReqOut) -> Mux/8
  ReqTrig8/1(ReqOut) -> Mux/9
  ReqTrig9/1(ReqOut) -> Mux/10
  ReqTrig10/1(ReqOut) -> Mux/11
  ReqTrig11/1(ReqOut) -> Mux/12
  ReqTrig12/1(ReqOut) -> Mux/13
  ReqTrig13/1(ReqOut) -> Mux/14
  ReqTrig14/1(ReqOut) -> Mux/15
  ReqTrig15/1(ReqOut) -> Mux/16
  ReqTrig16/1(ReqOut) -> Mux/17
  ReqTrig17/1(ReqOut) -> Mux/18
  ReqTrig18/1(ReqOut) -> Mux/19
  ReqTrig19/1(ReqOut) -> Mux/20
  ReqTrig20/1(ReqOut) -> Mux/21
  ReqTrig21/1(ReqOut) -> Mux/22
  ReqTrig22/1(ReqOut) -> Mux/23
  ReqTrig23/1(ReqOut) -> Mux/24
  Constant45/1 -> Bitwise Operator7/6
  Shift Arithmetic15/1 -> Bitwise Operator3/11
  Data Type Conversion49/1 -> Shift Arithmetic15/1
  Constant94/1 -> Data Type Conversion49/1
  LfFamlyReq_Val_read/1 -> Terminator/1
  RtFamlyMdReq_Val_read/1 -> Terminator1/1
  Md61MemReq_Val_read/1 -> Logical Operator8/1
  Md61Req_Val_read/1 -> Logical Operator8/2
  Md62Req_Val_read/1 -> Logical Operator9/2
  Md62MemReq_Val_read/1 -> Logical Operator9/1
  Logical Operator9/1 -> ReqTrig7/1(Req)
  Logical Operator8/1 -> ReqTrig8/1(Req)
  BigBedAllMdReq_Val_read/1 -> Logical Operator11/2
  Logical Operator10/1 -> Logical Operator11/1
  BigBedLMdAvl_Val_read/1 -> [BigBedLMdAvl], Logical Operator10/1
  BigBedRMdAvl_Val_read/1 -> [BigBedRMdAvl], Logical Operator10/2
  Logical Operator11/1 -> [BigBedAll]
  BigBedLtMdReq_Val_read/1 -> ReqTrig24/1(Req)
  ReqTrig24/1(ReqOut) -> Mux/25
  BigBedRtMdReq_Val_read/1 -> ReqTrig25/1(Req)
  ReqTrig25/1(ReqOut) -> Mux/26
  [BigBedAll] -> ReqTrig26/1(Req)
  ReqTrig26/1(ReqOut) -> Mux/27
  Ground/1 -> Mux/32, Mux/31, Mux/30, Mux/29, Mux/28
  Constant95/1 -> Mux2/25
  Constant96/1 -> Mux2/26
  Ground2/1 -> Mux2/28, Mux2/32, Mux2/31, Mux2/30, Mux2/29
  Shift Arithmetic78/1 -> Bitwise Operator15/3
  [BigBedRMdAvl] -> Data Type Conversion51/1
  Data Type Conversion50/1 -> Shift Arithmetic37/1
  Data Type Conversion51/1 -> Shift Arithmetic78/1
  Shift Arithmetic37/1 -> Bitwise Operator15/2
  [BigBedLMdAvl] -> Data Type Conversion50/1
  Constant98/1 -> Bitwise Operator15/1
  Bitwise Operator15/1 -> Mux2/27
  [LftBsyBitVIP] -> Mux3/25
  [RghtBsyBitVIP] -> Mux3/26
  Constant101/1 -> Mux3/27
  Ground3/1 -> Mux3/32, Mux3/31, Mux3/30, Mux3/29, Mux3/28
  Shift Arithmetic80/1 -> Bitwise Operator3/12
  Data Type Conversion53/1 -> Shift Arithmetic80/1
  Constant102/1 -> Data Type Conversion53/1
  [is7s] -> Data Type Conversion54/1
  Data Type Conversion54/1 -> Shift Arithmetic81/1
  Shift Arithmetic81/1 -> Bitwise Operator2/9  "bedl"

== system MdSWReqChk/MdSWReqChk_Cal_sys/Subsystem/ReqTrig ==
  Req : Inport
  Logical Operator : Logic  AllPortsSameDT=off  OutDataTypeStr=boolean
  Logical Operator1 : Logic  Operator=NOT  AllPortsSameDT=off  OutDataTypeStr=boolean
  Unit Delay : UnitDelay  SampleTime=-1  HasFrameUpgradeWarning=on
  ReqOut : Outport  VectorParamsAs1DForOutWhenUnconnected=off
  wires:
  Req/1 -> Logical Operator/1, Unit Delay/1
  Logical Operator/1 -> ReqOut/1
  Unit Delay/1 -> Logical Operator1/1
  Logical Operator1/1 -> Logical Operator/2

== system MdSWReqChk/MdSWReqChk_Cal_sys/Subsystem/ReqTrig1 ==
  Req : Inport
  Logical Operator : Logic  AllPortsSameDT=off  OutDataTypeStr=boolean
  Logical Operator1 : Logic  Operator=NOT  AllPortsSameDT=off  OutDataTypeStr=boolean
  Unit Delay : UnitDelay  SampleTime=-1  HasFrameUpgradeWarning=on
  ReqOut : Outport  VectorParamsAs1DForOutWhenUnconnected=off
  wires:
  Logical Operator1/1 -> Logical Operator/2
  Unit Delay/1 -> Logical Operator1/1
  Logical Operator/1 -> ReqOut/1
  Req/1 -> Unit Delay/1, Logical Operator/1

== system MdSWReqChk/MdSWReqChk_Cal_sys/Subsystem/ReqTrig10 ==
  Req : Inport
  Logical Operator : Logic  AllPortsSameDT=off  OutDataTypeStr=boolean
  Logical Operator1 : Logic  Operator=NOT  AllPortsSameDT=off  OutDataTypeStr=boolean
  Unit Delay : UnitDelay  SampleTime=-1  HasFrameUpgradeWarning=on
  ReqOut : Outport  VectorParamsAs1DForOutWhenUnconnected=off
  wires:
  Req/1 -> Logical Operator/1, Unit Delay/1
  Logical Operator/1 -> ReqOut/1
  Unit Delay/1 -> Logical Operator1/1
  Logical Operator1/1 -> Logical Operator/2

== system MdSWReqChk/MdSWReqChk_Cal_sys/Subsystem/ReqTrig11 ==
  Req : Inport
  Logical Operator : Logic  AllPortsSameDT=off  OutDataTypeStr=boolean
  Logical Operator1 : Logic  Operator=NOT  AllPortsSameDT=off  OutDataTypeStr=boolean
  Unit Delay : UnitDelay  SampleTime=-1  HasFrameUpgradeWarning=on
  ReqOut : Outport  VectorParamsAs1DForOutWhenUnconnected=off
  wires:
  Logical Operator1/1 -> Logical Operator/2
  Unit Delay/1 -> Logical Operator1/1
  Logical Operator/1 -> ReqOut/1
  Req/1 -> Unit Delay/1, Logical Operator/1

== system MdSWReqChk/MdSWReqChk_Cal_sys/Subsystem/ReqTrig12 ==
  Req : Inport
  Logical Operator : Logic  AllPortsSameDT=off  OutDataTypeStr=boolean
  Logical Operator1 : Logic  Operator=NOT  AllPortsSameDT=off  OutDataTypeStr=boolean
  Unit Delay : UnitDelay  SampleTime=-1  HasFrameUpgradeWarning=on
  ReqOut : Outport  VectorParamsAs1DForOutWhenUnconnected=off
  wires:
  Req/1 -> Logical Operator/1, Unit Delay/1
  Logical Operator/1 -> ReqOut/1
  Unit Delay/1 -> Logical Operator1/1
  Logical Operator1/1 -> Logical Operator/2

== system MdSWReqChk/MdSWReqChk_Cal_sys/Subsystem/ReqTrig13 ==
  Req : Inport
  Logical Operator : Logic  AllPortsSameDT=off  OutDataTypeStr=boolean
  Logical Operator1 : Logic  Operator=NOT  AllPortsSameDT=off  OutDataTypeStr=boolean
  Unit Delay : UnitDelay  SampleTime=-1  HasFrameUpgradeWarning=on
  ReqOut : Outport  VectorParamsAs1DForOutWhenUnconnected=off
  wires:
  Logical Operator1/1 -> Logical Operator/2
  Unit Delay/1 -> Logical Operator1/1
  Logical Operator/1 -> ReqOut/1
  Req/1 -> Unit Delay/1, Logical Operator/1

== system MdSWReqChk/MdSWReqChk_Cal_sys/Subsystem/ReqTrig14 ==
  Req : Inport
  Logical Operator : Logic  AllPortsSameDT=off  OutDataTypeStr=boolean
  Logical Operator1 : Logic  Operator=NOT  AllPortsSameDT=off  OutDataTypeStr=boolean
  Unit Delay : UnitDelay  SampleTime=-1  HasFrameUpgradeWarning=on
  ReqOut : Outport  VectorParamsAs1DForOutWhenUnconnected=off
  wires:
  Req/1 -> Logical Operator/1, Unit Delay/1
  Logical Operator/1 -> ReqOut/1
  Unit Delay/1 -> Logical Operator1/1
  Logical Operator1/1 -> Logical Operator/2

== system MdSWReqChk/MdSWReqChk_Cal_sys/Subsystem/ReqTrig15 ==
  Req : Inport
  Logical Operator : Logic  AllPortsSameDT=off  OutDataTypeStr=boolean
  Logical Operator1 : Logic  Operator=NOT  AllPortsSameDT=off  OutDataTypeStr=boolean
  Unit Delay : UnitDelay  SampleTime=-1  HasFrameUpgradeWarning=on
  ReqOut : Outport  VectorParamsAs1DForOutWhenUnconnected=off
  wires:
  Logical Operator1/1 -> Logical Operator/2
  Unit Delay/1 -> Logical Operator1/1
  Logical Operator/1 -> ReqOut/1
  Req/1 -> Unit Delay/1, Logical Operator/1

== system MdSWReqChk/MdSWReqChk_Cal_sys/Subsystem/ReqTrig16 ==
  Req : Inport
  Logical Operator : Logic  AllPortsSameDT=off  OutDataTypeStr=boolean
  Logical Operator1 : Logic  Operator=NOT  AllPortsSameDT=off  OutDataTypeStr=boolean
  Unit Delay : UnitDelay  SampleTime=-1  HasFrameUpgradeWarning=on
  ReqOut : Outport  VectorParamsAs1DForOutWhenUnconnected=off
  wires:
  Req/1 -> Logical Operator/1, Unit Delay/1
  Logical Operator/1 -> ReqOut/1
  Unit Delay/1 -> Logical Operator1/1
  Logical Operator1/1 -> Logical Operator/2

== system MdSWReqChk/MdSWReqChk_Cal_sys/Subsystem/ReqTrig17 ==
  Req : Inport
  Logical Operator : Logic  AllPortsSameDT=off  OutDataTypeStr=boolean
  Logical Operator1 : Logic  Operator=NOT  AllPortsSameDT=off  OutDataTypeStr=boolean
  Unit Delay : UnitDelay  SampleTime=-1  HasFrameUpgradeWarning=on
  ReqOut : Outport  VectorParamsAs1DForOutWhenUnconnected=off
  wires:
  Logical Operator1/1 -> Logical Operator/2
  Unit Delay/1 -> Logical Operator1/1
  Logical Operator/1 -> ReqOut/1
  Req/1 -> Unit Delay/1, Logical Operator/1

== system MdSWReqChk/MdSWReqChk_Cal_sys/Subsystem/ReqTrig18 ==
  Req : Inport
  Logical Operator : Logic  AllPortsSameDT=off  OutDataTypeStr=boolean
  Logical Operator1 : Logic  Operator=NOT  AllPortsSameDT=off  OutDataTypeStr=boolean
  Unit Delay : UnitDelay  SampleTime=-1  HasFrameUpgradeWarning=on
  ReqOut : Outport  VectorParamsAs1DForOutWhenUnconnected=off
  wires:
  Req/1 -> Logical Operator/1, Unit Delay/1
  Logical Operator/1 -> ReqOut/1
  Unit Delay/1 -> Logical Operator1/1
  Logical Operator1/1 -> Logical Operator/2

== system MdSWReqChk/MdSWReqChk_Cal_sys/Subsystem/ReqTrig19 ==
  Req : Inport
  Logical Operator : Logic  AllPortsSameDT=off  OutDataTypeStr=boolean
  Logical Operator1 : Logic  Operator=NOT  AllPortsSameDT=off  OutDataTypeStr=boolean
  Unit Delay : UnitDelay  SampleTime=-1  HasFrameUpgradeWarning=on
  ReqOut : Outport  VectorParamsAs1DForOutWhenUnconnected=off
  wires:
  Logical Operator1/1 -> Logical Operator/2
  Unit Delay/1 -> Logical Operator1/1
  Logical Operator/1 -> ReqOut/1
  Req/1 -> Unit Delay/1, Logical Operator/1

== system MdSWReqChk/MdSWReqChk_Cal_sys/Subsystem/ReqTrig2 ==
  Req : Inport
  Logical Operator : Logic  AllPortsSameDT=off  OutDataTypeStr=boolean
  Logical Operator1 : Logic  Operator=NOT  AllPortsSameDT=off  OutDataTypeStr=boolean
  Unit Delay : UnitDelay  SampleTime=-1  HasFrameUpgradeWarning=on
  ReqOut : Outport  VectorParamsAs1DForOutWhenUnconnected=off
  wires:
  Req/1 -> Logical Operator/1, Unit Delay/1
  Logical Operator/1 -> ReqOut/1
  Unit Delay/1 -> Logical Operator1/1
  Logical Operator1/1 -> Logical Operator/2

== system MdSWReqChk/MdSWReqChk_Cal_sys/Subsystem/ReqTrig20 ==
  Req : Inport
  Logical Operator : Logic  AllPortsSameDT=off  OutDataTypeStr=boolean
  Logical Operator1 : Logic  Operator=NOT  AllPortsSameDT=off  OutDataTypeStr=boolean
  Unit Delay : UnitDelay  SampleTime=-1  HasFrameUpgradeWarning=on
  ReqOut : Outport  VectorParamsAs1DForOutWhenUnconnected=off
  wires:
  Req/1 -> Logical Operator/1, Unit Delay/1
  Logical Operator/1 -> ReqOut/1
  Unit Delay/1 -> Logical Operator1/1
  Logical Operator1/1 -> Logical Operator/2

== system MdSWReqChk/MdSWReqChk_Cal_sys/Subsystem/ReqTrig21 ==
  Req : Inport
  Logical Operator : Logic  AllPortsSameDT=off  OutDataTypeStr=boolean
  Logical Operator1 : Logic  Operator=NOT  AllPortsSameDT=off  OutDataTypeStr=boolean
  Unit Delay : UnitDelay  SampleTime=-1  HasFrameUpgradeWarning=on
  ReqOut : Outport  VectorParamsAs1DForOutWhenUnconnected=off
  wires:
  Logical Operator1/1 -> Logical Operator/2
  Unit Delay/1 -> Logical Operator1/1
  Logical Operator/1 -> ReqOut/1
  Req/1 -> Unit Delay/1, Logical Operator/1

== system MdSWReqChk/MdSWReqChk_Cal_sys/Subsystem/ReqTrig22 ==
  Req : Inport
  Logical Operator : Logic  AllPortsSameDT=off  OutDataTypeStr=boolean
  Logical Operator1 : Logic  Operator=NOT  AllPortsSameDT=off  OutDataTypeStr=boolean
  Unit Delay : UnitDelay  SampleTime=-1  HasFrameUpgradeWarning=on
  ReqOut : Outport  VectorParamsAs1DForOutWhenUnconnected=off
  wires:
  Req/1 -> Logical Operator/1, Unit Delay/1
  Logical Operator/1 -> ReqOut/1
  Unit Delay/1 -> Logical Operator1/1
  Logical Operator1/1 -> Logical Operator/2

== system MdSWReqChk/MdSWReqChk_Cal_sys/Subsystem/ReqTrig23 ==
  Req : Inport
  Logical Operator : Logic  AllPortsSameDT=off  OutDataTypeStr=boolean
  Logical Operator1 : Logic  Operator=NOT  AllPortsSameDT=off  OutDataTypeStr=boolean
  Unit Delay : UnitDelay  SampleTime=-1  HasFrameUpgradeWarning=on
  ReqOut : Outport  VectorParamsAs1DForOutWhenUnconnected=off
  wires:
  Logical Operator1/1 -> Logical Operator/2
  Unit Delay/1 -> Logical Operator1/1
  Logical Operator/1 -> ReqOut/1
  Req/1 -> Unit Delay/1, Logical Operator/1

== system MdSWReqChk/MdSWReqChk_Cal_sys/Subsystem/ReqTrig24 ==
  Req : Inport
  Logical Operator : Logic  AllPortsSameDT=off  OutDataTypeStr=boolean
  Logical Operator1 : Logic  Operator=NOT  AllPortsSameDT=off  OutDataTypeStr=boolean
  Unit Delay : UnitDelay  SampleTime=-1  HasFrameUpgradeWarning=on
  ReqOut : Outport  VectorParamsAs1DForOutWhenUnconnected=off
  wires:
  Logical Operator1/1 -> Logical Operator/2
  Unit Delay/1 -> Logical Operator1/1
  Logical Operator/1 -> ReqOut/1
  Req/1 -> Unit Delay/1, Logical Operator/1

== system MdSWReqChk/MdSWReqChk_Cal_sys/Subsystem/ReqTrig25 ==
  Req : Inport
  Logical Operator : Logic  AllPortsSameDT=off  OutDataTypeStr=boolean
  Logical Operator1 : Logic  Operator=NOT  AllPortsSameDT=off  OutDataTypeStr=boolean
  Unit Delay : UnitDelay  SampleTime=-1  HasFrameUpgradeWarning=on
  ReqOut : Outport  VectorParamsAs1DForOutWhenUnconnected=off
  wires:
  Logical Operator1/1 -> Logical Operator/2
  Unit Delay/1 -> Logical Operator1/1
  Logical Operator/1 -> ReqOut/1
  Req/1 -> Unit Delay/1, Logical Operator/1

== system MdSWReqChk/MdSWReqChk_Cal_sys/Subsystem/ReqTrig26 ==
  Req : Inport
  Logical Operator : Logic  AllPortsSameDT=off  OutDataTypeStr=boolean
  Logical Operator1 : Logic  Operator=NOT  AllPortsSameDT=off  OutDataTypeStr=boolean
  Unit Delay : UnitDelay  SampleTime=-1  HasFrameUpgradeWarning=on
  ReqOut : Outport  VectorParamsAs1DForOutWhenUnconnected=off
  wires:
  Logical Operator1/1 -> Logical Operator/2
  Unit Delay/1 -> Logical Operator1/1
  Logical Operator/1 -> ReqOut/1
  Req/1 -> Unit Delay/1, Logical Operator/1

== system MdSWReqChk/MdSWReqChk_Cal_sys/Subsystem/ReqTrig3 ==
  Req : Inport
  Logical Operator : Logic  AllPortsSameDT=off  OutDataTypeStr=boolean
  Logical Operator1 : Logic  Operator=NOT  AllPortsSameDT=off  OutDataTypeStr=boolean
  Unit Delay : UnitDelay  SampleTime=-1  HasFrameUpgradeWarning=on
  ReqOut : Outport  VectorParamsAs1DForOutWhenUnconnected=off
  wires:
  Logical Operator1/1 -> Logical Operator/2
  Unit Delay/1 -> Logical Operator1/1
  Logical Operator/1 -> ReqOut/1
  Req/1 -> Unit Delay/1, Logical Operator/1

== system MdSWReqChk/MdSWReqChk_Cal_sys/Subsystem/ReqTrig4 ==
  Req : Inport
  Logical Operator : Logic  AllPortsSameDT=off  OutDataTypeStr=boolean
  Logical Operator1 : Logic  Operator=NOT  AllPortsSameDT=off  OutDataTypeStr=boolean
  Unit Delay : UnitDelay  SampleTime=-1  HasFrameUpgradeWarning=on
  ReqOut : Outport  VectorParamsAs1DForOutWhenUnconnected=off
  wires:
  Req/1 -> Logical Operator/1, Unit Delay/1
  Logical Operator/1 -> ReqOut/1
  Unit Delay/1 -> Logical Operator1/1
  Logical Operator1/1 -> Logical Operator/2

== system MdSWReqChk/MdSWReqChk_Cal_sys/Subsystem/ReqTrig5 ==
  Req : Inport
  Logical Operator : Logic  AllPortsSameDT=off  OutDataTypeStr=boolean
  Logical Operator1 : Logic  Operator=NOT  AllPortsSameDT=off  OutDataTypeStr=boolean
  Unit Delay : UnitDelay  SampleTime=-1  HasFrameUpgradeWarning=on
  ReqOut : Outport  VectorParamsAs1DForOutWhenUnconnected=off
  wires:
  Logical Operator1/1 -> Logical Operator/2
  Unit Delay/1 -> Logical Operator1/1
  Logical Operator/1 -> ReqOut/1
  Req/1 -> Unit Delay/1, Logical Operator/1

== system MdSWReqChk/MdSWReqChk_Cal_sys/Subsystem/ReqTrig6 ==
  Req : Inport
  Logical Operator : Logic  AllPortsSameDT=off  OutDataTypeStr=boolean
  Logical Operator1 : Logic  Operator=NOT  AllPortsSameDT=off  OutDataTypeStr=boolean
  Unit Delay : UnitDelay  SampleTime=-1  HasFrameUpgradeWarning=on
  ReqOut : Outport  VectorParamsAs1DForOutWhenUnconnected=off
  wires:
  Req/1 -> Logical Operator/1, Unit Delay/1
  Logical Operator/1 -> ReqOut/1
  Unit Delay/1 -> Logical Operator1/1
  Logical Operator1/1 -> Logical Operator/2

== system MdSWReqChk/MdSWReqChk_Cal_sys/Subsystem/ReqTrig7 ==
  Req : Inport
  Logical Operator : Logic  AllPortsSameDT=off  OutDataTypeStr=boolean
  Logical Operator1 : Logic  Operator=NOT  AllPortsSameDT=off  OutDataTypeStr=boolean
  Unit Delay : UnitDelay  SampleTime=-1  HasFrameUpgradeWarning=on
  ReqOut : Outport  VectorParamsAs1DForOutWhenUnconnected=off
  wires:
  Logical Operator1/1 -> Logical Operator/2
  Unit Delay/1 -> Logical Operator1/1
  Logical Operator/1 -> ReqOut/1
  Req/1 -> Unit Delay/1, Logical Operator/1

== system MdSWReqChk/MdSWReqChk_Cal_sys/Subsystem/ReqTrig8 ==
  Req : Inport
  Logical Operator : Logic  AllPortsSameDT=off  OutDataTypeStr=boolean
  Logical Operator1 : Logic  Operator=NOT  AllPortsSameDT=off  OutDataTypeStr=boolean
  Unit Delay : UnitDelay  SampleTime=-1  HasFrameUpgradeWarning=on
  ReqOut : Outport  VectorParamsAs1DForOutWhenUnconnected=off
  wires:
  Req/1 -> Logical Operator/1, Unit Delay/1
  Logical Operator/1 -> ReqOut/1
  Unit Delay/1 -> Logical Operator1/1
  Logical Operator1/1 -> Logical Operator/2

== system MdSWReqChk/MdSWReqChk_Cal_sys/Subsystem/ReqTrig9 ==
  Req : Inport
  Logical Operator : Logic  AllPortsSameDT=off  OutDataTypeStr=boolean
  Logical Operator1 : Logic  Operator=NOT  AllPortsSameDT=off  OutDataTypeStr=boolean
  Unit Delay : UnitDelay  SampleTime=-1  HasFrameUpgradeWarning=on
  ReqOut : Outport  VectorParamsAs1DForOutWhenUnconnected=off
  wires:
  Logical Operator1/1 -> Logical Operator/2
  Unit Delay/1 -> Logical Operator1/1
  Logical Operator/1 -> ReqOut/1
  Req/1 -> Unit Delay/1, Logical Operator/1
